simulink model "cla64bit"  (R2020a)
settings: Solver=VariableStepAuto  StartTime=0.0  StopTime=10.0  RelTol=1e-3
(part 1 of 3)
settings Model: Creator=kishan  LastModifiedBy=kishan

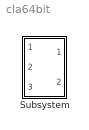
== system cla64bit ==
  Subsystem : Subsystem

== system cla64bit/Subsystem ==
  In1 : Inport
  In3 : Inport  Port=2
  In2 : Inport  Port=3
  Demux : Demux  Outputs=2
  Demux1 : Demux  Outputs=2
  Mux : Mux  Inputs=2
  Subsystem1 : Subsystem
  Subsystem8 : Subsystem
  Out1 : Outport
  Out2 : Outport  Port=2
  wires:
  In1/1 -> Demux/1
  Subsystem8/1(Out1) -> Subsystem1/2(In1)
  Demux1/1 -> Subsystem1/3(In3)
  Mux/1 -> Out2/1
  Subsystem1/1(Out1) -> Out1/1
  Subsystem8/2(Out2) -> Mux/2
  Demux/1 -> Subsystem1/1(In2)
  Demux/2 -> Subsystem8/1(In2)
  Demux1/2 -> Subsystem8/3(In3)
  Subsystem1/2(Out2) -> Mux/1
  In3/1 -> Subsystem8/2(In1)
  In2/1 -> Demux1/1

== system cla64bit/Subsystem/Subsystem1 ==
  In2 : Inport
  In1 : Inport  Port=2
  In3 : Inport  Port=3
  Demux : Demux  Outputs=32
  Demux1 : Demux  Outputs=32
  Mux : Mux  Inputs=32
  Subsystem : Subsystem
  Subsystem1 : Subsystem
  Subsystem2 : Subsystem
  Subsystem3 : Subsystem
  Subsystem4 : Subsystem
  Subsystem5 : Subsystem
  Subsystem6 : Subsystem
  Subsystem7 : Subsystem
  Out1 : Outport
  Out2 : Outport  Port=2
  wires:
  Demux1/30 -> Subsystem/7(In7)
  Demux/11 -> Subsystem5/3(In3)
  Subsystem4/4(Out4) -> Mux/15
  Demux/29 -> Subsystem/1(In1)
  Demux1/4 -> Subsystem7/9(In9)
  Demux/14 -> Subsystem4/2(In2)
  Subsystem/2(Out2) -> Mux/29
  Subsystem7/4(Out4) -> Mux/3
  Subsystem2/3(Out3) -> Mux/22
  Demux/26 -> Subsystem1/2(In2)
  Subsystem7/1(Out1) -> Out1/1
  Subsystem7/3(Out3) -> Mux/2
  Demux/3 -> Subsystem7/3(In3)
  Demux/15 -> Subsystem4/3(In3)
  Subsystem6/1(Out1) -> Subsystem7/5(In5)
  In3/1 -> Demux1/1
  Demux1/31 -> Subsystem/8(In8)
  Demux/20 -> Subsystem3/4(In4)
  Subsystem4/5(Out5) -> Mux/16
  Demux/19 -> Subsystem3/3(In3)
  Subsystem3/5(Out5) -> Mux/20
  Demux1/22 -> Subsystem2/7(In7)
  Subsystem4/3(Out3) -> Mux/14
  Subsystem1/2(Out2) -> Mux/25
  Demux1/15 -> Subsystem4/8(In8)
  Subsystem/4(Out4) -> Mux/31
  Demux/24 -> Subsystem2/4(In4)
  Subsystem5/4(Out4) -> Mux/11
  Subsystem3/3(Out3) -> Mux/18
  Subsystem5/1(Out1) -> Subsystem6/5(In5)
  Subsystem2/2(Out2) -> Mux/21
  Subsystem5/3(Out3) -> Mux/10
  Demux1/16 -> Subsystem4/9(In9)
  Demux/9 -> Subsystem5/1(In1)
  Subsystem7/5(Out5) -> Mux/4
  Demux1/3 -> Subsystem7/8(In8)
  Demux1/29 -> Subsystem/6(In6)
  Demux1/9 -> Subsystem5/6(In6)
  Subsystem2/1(Out1) -> Subsystem3/5(In5)
  Subsystem6/5(Out5) -> Mux/8
  Demux1/25 -> Subsystem1/6(In6)
  Demux/1 -> Subsystem7/1(In1)
  Demux1/13 -> Subsystem4/6(In6)
  Demux/5 -> Subsystem6/1(In1)
  Demux1/7 -> Subsystem6/8(In8)
  Demux1/20 -> Subsystem3/9(In9)
  Subsystem1/4(Out4) -> Mux/27
  In2/1 -> Demux/1
  Demux1/12 -> Subsystem5/9(In9)
  Demux1/18 -> Subsystem3/7(In7)
  Demux/22 -> Subsystem2/2(In2)
  Demux1/32 -> Subsystem/9(In9)
  Subsystem2/4(Out4) -> Mux/23
  Subsystem6/4(Out4) -> Mux/7
  Subsystem5/5(Out5) -> Mux/12
  Demux1/23 -> Subsystem2/8(In8)
  Mux/1 -> Out2/1
  Subsystem6/3(Out3) -> Mux/6
  Demux1/8 -> Subsystem6/9(In9)
  In1/1 -> Subsystem/5(In5)
  Demux/12 -> Subsystem5/4(In4)
  Demux1/17 -> Subsystem3/6(In6)
  Subsystem1/1(Out1) -> Subsystem2/5(In5)
  Subsystem1/5(Out5) -> Mux/28
  Subsystem4/1(Out1) -> Subsystem5/5(In5)
  Demux/6 -> Subsystem6/2(In2)
  Subsystem6/2(Out2) -> Mux/5
  Demux/25 -> Subsystem1/1(In1)
  Subsystem/5(Out5) -> Mux/32
  Subsystem1/3(Out3) -> Mux/26
  Demux1/1 -> Subsystem7/6(In6)
  Demux/31 -> Subsystem/3(In3)
  Demux1/26 -> Subsystem1/7(In7)
  Subsystem/3(Out3) -> Mux/30
  Subsystem3/1(Out1) -> Subsystem4/5(In5)
  Demux/8 -> Subsystem6/4(In4)
  Demux/32 -> Subsystem/4(In4)
  Demux1/19 -> Subsystem3/8(In8)
  Demux1/5 -> Subsystem6/6(In6)
  Subsystem3/4(Out4) -> Mux/19
  Demux/27 -> Subsystem1/3(In3)
  Subsystem/1(Out1) -> Subsystem1/5(In5)
  Demux1/24 -> Subsystem2/9(In9)
  Demux/7 -> Subsystem6/3(In3)
  Demux/30 -> Subsystem/2(In2)
  Demux/4 -> Subsystem7/4(In4)
  Demux/10 -> Subsystem5/2(In2)
  Demux1/28 -> Subsystem1/9(In9)
  Subsystem5/2(Out2) -> Mux/9
  Demux/2 -> Subsystem7/2(In2)
  Demux/17 -> Subsystem3/1(In1)
  Subsystem2/5(Out5) -> Mux/24
  Demux1/6 -> Subsystem6/7(In7)
  Subsystem7/2(Out2) -> Mux/1
  Subsystem4/2(Out2) -> Mux/13
  Demux/13 -> Subsystem4/1(In1)
  Demux/21 -> Subsystem2/1(In1)
  Demux/18 -> Subsystem3/2(In2)
  Subsystem3/2(Out2) -> Mux/17
  Demux1/27 -> Subsystem1/8(In8)
  Demux1/11 -> Subsystem5/8(In8)
  Demux/28 -> Subsystem1/4(In4)
  Demux1/2 -> Subsystem7/7(In7)
  Demux/23 -> Subsystem2/3(In3)
  Demux1/21 -> Subsystem2/6(In6)
  Demux1/14 -> Subsystem4/7(In7)
  Demux/16 -> Subsystem4/4(In4)
  Demux1/10 -> Subsystem5/7(In7)

== system cla64bit/Subsystem/Subsystem8 ==
  In2 : Inport
  In1 : Inport  Port=2
  In3 : Inport  Port=3
  Demux : Demux  Outputs=32
  Demux1 : Demux  Outputs=32
  Mux : Mux  Inputs=32
  Subsystem : Subsystem
  Subsystem1 : Subsystem
  Subsystem2 : Subsystem
  Subsystem3 : Subsystem
  Subsystem4 : Subsystem
  Subsystem5 : Subsystem
  Subsystem6 : Subsystem
  Subsystem7 : Subsystem
  Out1 : Outport
  Out2 : Outport  Port=2
  wires:
  Demux1/30 -> Subsystem/7(In7)
  Demux/11 -> Subsystem5/3(In3)
  Subsystem4/4(Out4) -> Mux/15
  Demux/29 -> Subsystem/1(In1)
  Demux1/4 -> Subsystem7/9(In9)
  Demux/14 -> Subsystem4/2(In2)
  Subsystem/2(Out2) -> Mux/29
  Subsystem7/4(Out4) -> Mux/3
  Subsystem2/3(Out3) -> Mux/22
  Demux/26 -> Subsystem1/2(In2)
  Subsystem7/1(Out1) -> Out1/1
  Subsystem7/3(Out3) -> Mux/2
  Demux/3 -> Subsystem7/3(In3)
  Demux/15 -> Subsystem4/3(In3)
  Subsystem6/1(Out1) -> Subsystem7/5(In5)
  In3/1 -> Demux1/1
  Demux1/31 -> Subsystem/8(In8)
  Demux/20 -> Subsystem3/4(In4)
  Subsystem4/5(Out5) -> Mux/16
  Demux/19 -> Subsystem3/3(In3)
  Subsystem3/5(Out5) -> Mux/20
  Demux1/22 -> Subsystem2/7(In7)
  Subsystem4/3(Out3) -> Mux/14
  Subsystem1/2(Out2) -> Mux/25
  Demux1/15 -> Subsystem4/8(In8)
  Subsystem/4(Out4) -> Mux/31
  Demux/24 -> Subsystem2/4(In4)
  Subsystem5/4(Out4) -> Mux/11
  Subsystem3/3(Out3) -> Mux/18
  Subsystem5/1(Out1) -> Subsystem6/5(In5)
  Subsystem2/2(Out2) -> Mux/21
  Subsystem5/3(Out3) -> Mux/10
  Demux1/16 -> Subsystem4/9(In9)
  Demux/9 -> Subsystem5/1(In1)
  Subsystem7/5(Out5) -> Mux/4
  Demux1/3 -> Subsystem7/8(In8)
  Demux1/29 -> Subsystem/6(In6)
  Demux1/9 -> Subsystem5/6(In6)
  Subsystem2/1(Out1) -> Subsystem3/5(In5)
  Subsystem6/5(Out5) -> Mux/8
  Demux1/25 -> Subsystem1/6(In6)
  Demux/1 -> Subsystem7/1(In1)
  Demux1/13 -> Subsystem4/6(In6)
  Demux/5 -> Subsystem6/1(In1)
  Demux1/7 -> Subsystem6/8(In8)
  Demux1/20 -> Subsystem3/9(In9)
  Subsystem1/4(Out4) -> Mux/27
  In2/1 -> Demux/1
  Demux1/12 -> Subsystem5/9(In9)
  Demux1/18 -> Subsystem3/7(In7)
  Demux/22 -> Subsystem2/2(In2)
  Demux1/32 -> Subsystem/9(In9)
  Subsystem2/4(Out4) -> Mux/23
  Subsystem6/4(Out4) -> Mux/7
  Subsystem5/5(Out5) -> Mux/12
  Demux1/23 -> Subsystem2/8(In8)
  Mux/1 -> Out2/1
  Subsystem6/3(Out3) -> Mux/6
  Demux1/8 -> Subsystem6/9(In9)
  In1/1 -> Subsystem/5(In5)
  Demux/12 -> Subsystem5/4(In4)
  Demux1/17 -> Subsystem3/6(In6)
  Subsystem1/1(Out1) -> Subsystem2/5(In5)
  Subsystem1/5(Out5) -> Mux/28
  Subsystem4/1(Out1) -> Subsystem5/5(In5)
  Demux/6 -> Subsystem6/2(In2)
  Subsystem6/2(Out2) -> Mux/5
  Demux/25 -> Subsystem1/1(In1)
  Subsystem/5(Out5) -> Mux/32
  Subsystem1/3(Out3) -> Mux/26
  Demux1/1 -> Subsystem7/6(In6)
  Demux/31 -> Subsystem/3(In3)
  Demux1/26 -> Subsystem1/7(In7)
  Subsystem/3(Out3) -> Mux/30
  Subsystem3/1(Out1) -> Subsystem4/5(In5)
  Demux/8 -> Subsystem6/4(In4)
  Demux/32 -> Subsystem/4(In4)
  Demux1/19 -> Subsystem3/8(In8)
  Demux1/5 -> Subsystem6/6(In6)
  Subsystem3/4(Out4) -> Mux/19
  Demux/27 -> Subsystem1/3(In3)
  Subsystem/1(Out1) -> Subsystem1/5(In5)
  Demux1/24 -> Subsystem2/9(In9)
  Demux/7 -> Subsystem6/3(In3)
  Demux/30 -> Subsystem/2(In2)
  Demux/4 -> Subsystem7/4(In4)
  Demux/10 -> Subsystem5/2(In2)
  Demux1/28 -> Subsystem1/9(In9)
  Subsystem5/2(Out2) -> Mux/9
  Demux/2 -> Subsystem7/2(In2)
  Demux/17 -> Subsystem3/1(In1)
  Subsystem2/5(Out5) -> Mux/24
  Demux1/6 -> Subsystem6/7(In7)
  Subsystem7/2(Out2) -> Mux/1
  Subsystem4/2(Out2) -> Mux/13
  Demux/13 -> Subsystem4/1(In1)
  Demux/21 -> Subsystem2/1(In1)
  Demux/18 -> Subsystem3/2(In2)
  Subsystem3/2(Out2) -> Mux/17
  Demux1/27 -> Subsystem1/8(In8)
  Demux1/11 -> Subsystem5/8(In8)
  Demux/28 -> Subsystem1/4(In4)
  Demux1/2 -> Subsystem7/7(In7)
  Demux/23 -> Subsystem2/3(In3)
  Demux1/21 -> Subsystem2/6(In6)
  Demux1/14 -> Subsystem4/7(In7)
  Demux/16 -> Subsystem4/4(In4)
  Demux1/10 -> Subsystem5/7(In7)

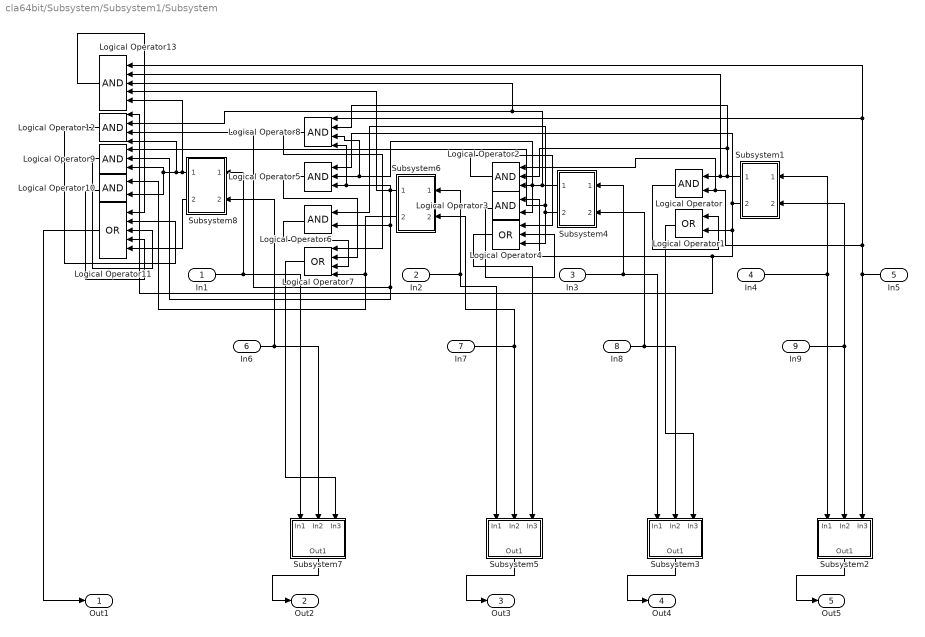
== system cla64bit/Subsystem/Subsystem1/Subsystem ==
  In1 : Inport
  In2 : Inport  Port=2
  In3 : Inport  Port=3
  In4 : Inport  Port=4
  In5 : Inport  Port=5
  In6 : Inport  Port=6
  In7 : Inport  Port=7
  In8 : Inport  Port=8
  In9 : Inport  Port=9
  Logical Operator{,3,6,10} (4 alike) : Logic  AllPortsSameDT=off  OutDataTypeStr=boolean
  Logical Operator1 : Logic  Operator=OR  AllPortsSameDT=off  OutDataTypeStr=boolean
  Logical Operator11 : Logic  Operator=OR  Inputs=5  AllPortsSameDT=off  OutDataTypeStr=boolean
  Logical Operator12 : Logic  Inputs=4  AllPortsSameDT=off  OutDataTypeStr=boolean
  Logical Operator13 : Logic  Inputs=5  AllPortsSameDT=off  OutDataTypeStr=boolean
  Logical Operator2 : Logic  Inputs=3  AllPortsSameDT=off  OutDataTypeStr=boolean
  Logical Operator4 : Logic  Operator=OR  Inputs=3  AllPortsSameDT=off  OutDataTypeStr=boolean
  Logical Operator5 : Logic  Inputs=3  AllPortsSameDT=off  OutDataTypeStr=boolean
  Logical Operator7 : Logic  Operator=OR  Inputs=4  AllPortsSameDT=off  OutDataTypeStr=boolean
  Logical Operator8 : Logic  Inputs=4  AllPortsSameDT=off  OutDataTypeStr=boolean
  Logical Operator9 : Logic  Inputs=3  AllPortsSameDT=off  OutDataTypeStr=boolean
  Subsystem1 : Subsystem
  Subsystem2 : Subsystem
  Subsystem3 : Subsystem
  Subsystem4 : Subsystem
  Subsystem5 : Subsystem
  Subsystem6 : Subsystem
  Subsystem7 : Subsystem
  Subsystem8 : Subsystem
  Out1 : Outport
  Out2 : Outport  Port=2
  Out3 : Outport  Port=3
  Out4 : Outport  Port=4
  Out5 : Outport  Port=5
  wires:
  Subsystem8/2(Out2) -> Logical Operator11/5
  Subsystem5/1(Out1) -> Out3/1
  Logical Operator8/1 -> Logical Operator7/1
  Logical Operator9/1 -> Logical Operator11/3
  Logical Operator5/1 -> Logical Operator7/2
  Logical Operator10/1 -> Logical Operator11/4
  Logical Operator3/1 -> Logical Operator4/2
  Logical Operator/1 -> Logical Operator1/1
  In3/1 -> Subsystem3/1(In1), Subsystem4/1(In1)
  Subsystem6/2(Out2) -> Logical Operator10/1, Logical Operator7/4
  Logical Operator12/1 -> Logical Operator11/2
  In7/1 -> Subsystem5/2(In2), Subsystem6/2(In2)
  Subsystem2/1(Out1) -> Out5/1
  In1/1 -> Subsystem8/1(In1), Subsystem7/1(In1)
  In6/1 -> Subsystem7/2(In2), Subsystem8/2(In2)
  Subsystem1/1(Out1) -> Logical Operator8/2, Logical Operator2/2, Logical Operator13/2, Logical Operator/1
  In9/1 -> Subsystem2/2(In2), Subsystem1/2(In2)
  In8/1 -> Subsystem3/2(In2), Subsystem4/2(In2)
  Logical Operator11/1 -> Out1/1
  Logical Operator2/1 -> Logical Operator4/1
  Subsystem4/1(Out1) -> Logical Operator8/3, Logical Operator5/2, Logical Operator3/2, Logical Operator2/3, Logical Operator13/3, Logical Operator12/2
  Logical Operator13/1 -> Logical Operator11/1
  Subsystem3/1(Out1) -> Out4/1
  In2/1 -> Subsystem6/1(In1), Subsystem5/1(In1)
  Logical Operator6/1 -> Logical Operator7/3
  Subsystem6/1(Out1) -> Logical Operator13/4, Logical Operator12/3, Logical Operator9/2, Logical Operator6/2, Logical Operator8/4, Logical Operator5/3
  Logical Operator7/1 -> Subsystem7/3(In3)
  Subsystem1/2(Out2) -> Logical Operator12/1, Logical Operator3/1, Logical Operator1/2, Logical Operator5/1
  In5/1 -> Subsystem2/3(In3), Logical Operator13/1, Logical Operator8/1, Logical Operator2/1, Logical Operator/2
  In4/1 -> Subsystem2/1(In1), Subsystem1/1(In1)
  Subsystem8/1(Out1) -> Logical Operator13/5, Logical Operator12/4, Logical Operator10/2, Logical Operator9/3
  Subsystem7/1(Out1) -> Out2/1
  Subsystem4/2(Out2) -> Logical Operator9/1, Logical Operator6/1, Logical Operator4/3
  Logical Operator4/1 -> Subsystem5/3(In3)
  Logical Operator1/1 -> Subsystem3/3(In3)

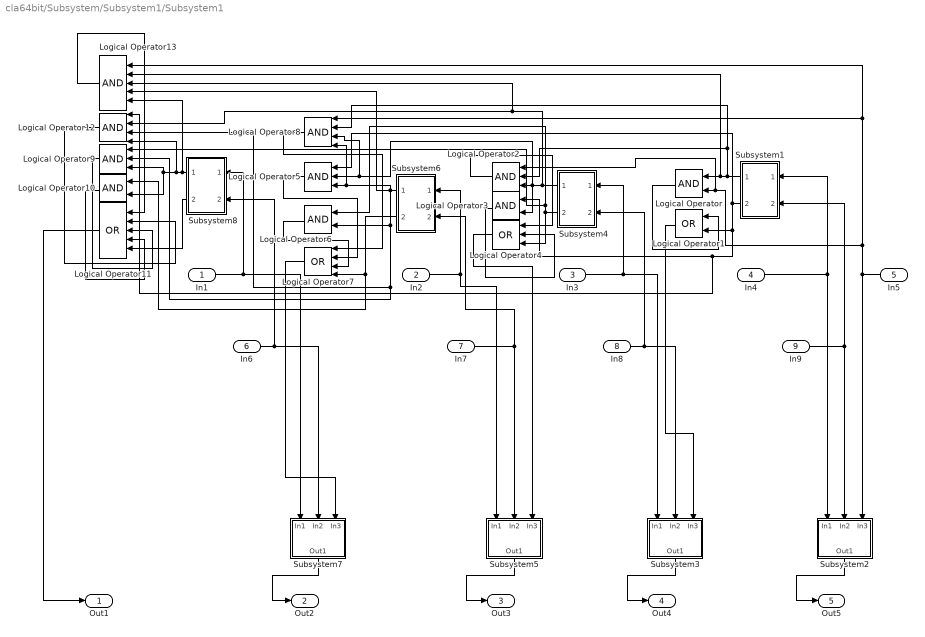
== system cla64bit/Subsystem/Subsystem1/Subsystem1 ==
  In1 : Inport
  In2 : Inport  Port=2
  In3 : Inport  Port=3
  In4 : Inport  Port=4
  In5 : Inport  Port=5
  In6 : Inport  Port=6
  In7 : Inport  Port=7
  In8 : Inport  Port=8
  In9 : Inport  Port=9
  Logical Operator{,3,6,10} (4 alike) : Logic  AllPortsSameDT=off  OutDataTypeStr=boolean
  Logical Operator1 : Logic  Operator=OR  AllPortsSameDT=off  OutDataTypeStr=boolean
  Logical Operator11 : Logic  Operator=OR  Inputs=5  AllPortsSameDT=off  OutDataTypeStr=boolean
  Logical Operator12 : Logic  Inputs=4  AllPortsSameDT=off  OutDataTypeStr=boolean
  Logical Operator13 : Logic  Inputs=5  AllPortsSameDT=off  OutDataTypeStr=boolean
  Logical Operator2 : Logic  Inputs=3  AllPortsSameDT=off  OutDataTypeStr=boolean
  Logical Operator4 : Logic  Operator=OR  Inputs=3  AllPortsSameDT=off  OutDataTypeStr=boolean
  Logical Operator5 : Logic  Inputs=3  AllPortsSameDT=off  OutDataTypeStr=boolean
  Logical Operator7 : Logic  Operator=OR  Inputs=4  AllPortsSameDT=off  OutDataTypeStr=boolean
  Logical Operator8 : Logic  Inputs=4  AllPortsSameDT=off  OutDataTypeStr=boolean
  Logical Operator9 : Logic  Inputs=3  AllPortsSameDT=off  OutDataTypeStr=boolean
  Subsystem1 : Subsystem
  Subsystem2 : Subsystem
  Subsystem3 : Subsystem
  Subsystem4 : Subsystem
  Subsystem5 : Subsystem
  Subsystem6 : Subsystem
  Subsystem7 : Subsystem
  Subsystem8 : Subsystem
  Out1 : Outport
  Out2 : Outport  Port=2
  Out3 : Outport  Port=3
  Out4 : Outport  Port=4
  Out5 : Outport  Port=5
  wires:
  Subsystem8/2(Out2) -> Logical Operator11/5
  Subsystem5/1(Out1) -> Out3/1
  Logical Operator8/1 -> Logical Operator7/1
  Logical Operator9/1 -> Logical Operator11/3
  Logical Operator5/1 -> Logical Operator7/2
  Logical Operator10/1 -> Logical Operator11/4
  Logical Operator3/1 -> Logical Operator4/2
  Logical Operator/1 -> Logical Operator1/1
  In3/1 -> Subsystem3/1(In1), Subsystem4/1(In1)
  Subsystem6/2(Out2) -> Logical Operator10/1, Logical Operator7/4
  Logical Operator12/1 -> Logical Operator11/2
  In7/1 -> Subsystem5/2(In2), Subsystem6/2(In2)
  Subsystem2/1(Out1) -> Out5/1
  In1/1 -> Subsystem8/1(In1), Subsystem7/1(In1)
  In6/1 -> Subsystem7/2(In2), Subsystem8/2(In2)
  Subsystem1/1(Out1) -> Logical Operator8/2, Logical Operator2/2, Logical Operator13/2, Logical Operator/1
  In9/1 -> Subsystem2/2(In2), Subsystem1/2(In2)
  In8/1 -> Subsystem3/2(In2), Subsystem4/2(In2)
  Logical Operator11/1 -> Out1/1
  Logical Operator2/1 -> Logical Operator4/1
  Subsystem4/1(Out1) -> Logical Operator8/3, Logical Operator5/2, Logical Operator3/2, Logical Operator2/3, Logical Operator13/3, Logical Operator12/2
  Logical Operator13/1 -> Logical Operator11/1
  Subsystem3/1(Out1) -> Out4/1
  In2/1 -> Subsystem6/1(In1), Subsystem5/1(In1)
  Logical Operator6/1 -> Logical Operator7/3
  Subsystem6/1(Out1) -> Logical Operator13/4, Logical Operator12/3, Logical Operator9/2, Logical Operator6/2, Logical Operator8/4, Logical Operator5/3
  Logical Operator7/1 -> Subsystem7/3(In3)
  Subsystem1/2(Out2) -> Logical Operator12/1, Logical Operator3/1, Logical Operator1/2, Logical Operator5/1
  In5/1 -> Subsystem2/3(In3), Logical Operator13/1, Logical Operator8/1, Logical Operator2/1, Logical Operator/2
  In4/1 -> Subsystem2/1(In1), Subsystem1/1(In1)
  Subsystem8/1(Out1) -> Logical Operator13/5, Logical Operator12/4, Logical Operator10/2, Logical Operator9/3
  Subsystem7/1(Out1) -> Out2/1
  Subsystem4/2(Out2) -> Logical Operator9/1, Logical Operator6/1, Logical Operator4/3
  Logical Operator4/1 -> Subsystem5/3(In3)
  Logical Operator1/1 -> Subsystem3/3(In3)

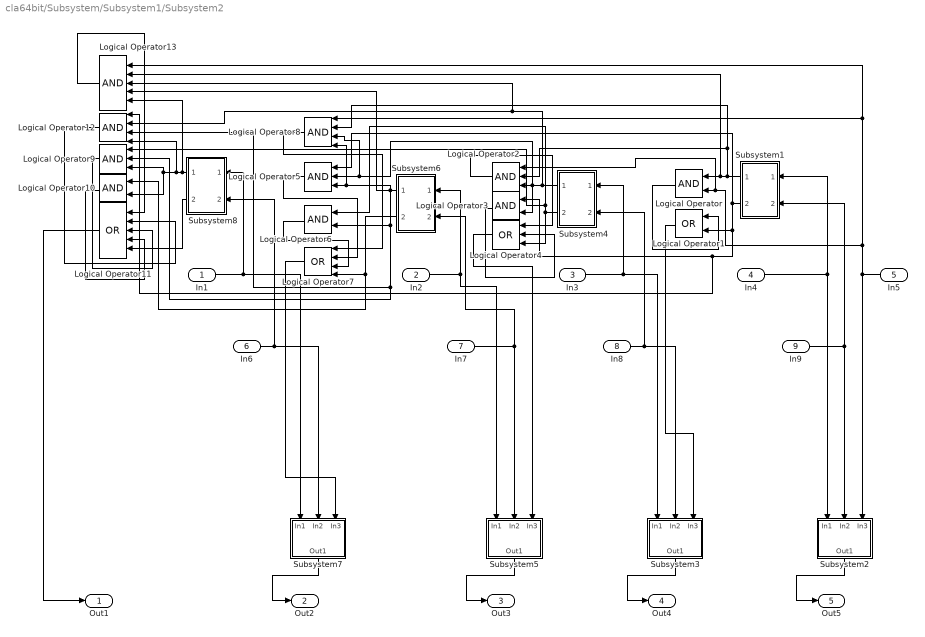
== system cla64bit/Subsystem/Subsystem1/Subsystem2 ==
  In1 : Inport
  In2 : Inport  Port=2
  In3 : Inport  Port=3
  In4 : Inport  Port=4
  In5 : Inport  Port=5
  In6 : Inport  Port=6
  In7 : Inport  Port=7
  In8 : Inport  Port=8
  In9 : Inport  Port=9
  Logical Operator{,3,6,10} (4 alike) : Logic  AllPortsSameDT=off  OutDataTypeStr=boolean
  Logical Operator1 : Logic  Operator=OR  AllPortsSameDT=off  OutDataTypeStr=boolean
  Logical Operator11 : Logic  Operator=OR  Inputs=5  AllPortsSameDT=off  OutDataTypeStr=boolean
  Logical Operator12 : Logic  Inputs=4  AllPortsSameDT=off  OutDataTypeStr=boolean
  Logical Operator13 : Logic  Inputs=5  AllPortsSameDT=off  OutDataTypeStr=boolean
  Logical Operator2 : Logic  Inputs=3  AllPortsSameDT=off  OutDataTypeStr=boolean
  Logical Operator4 : Logic  Operator=OR  Inputs=3  AllPortsSameDT=off  OutDataTypeStr=boolean
  Logical Operator5 : Logic  Inputs=3  AllPortsSameDT=off  OutDataTypeStr=boolean
  Logical Operator7 : Logic  Operator=OR  Inputs=4  AllPortsSameDT=off  OutDataTypeStr=boolean
  Logical Operator8 : Logic  Inputs=4  AllPortsSameDT=off  OutDataTypeStr=boolean
  Logical Operator9 : Logic  Inputs=3  AllPortsSameDT=off  OutDataTypeStr=boolean
  Subsystem1 : Subsystem
  Subsystem2 : Subsystem
  Subsystem3 : Subsystem
  Subsystem4 : Subsystem
  Subsystem5 : Subsystem
  Subsystem6 : Subsystem
  Subsystem7 : Subsystem
  Subsystem8 : Subsystem
  Out1 : Outport
  Out2 : Outport  Port=2
  Out3 : Outport  Port=3
  Out4 : Outport  Port=4
  Out5 : Outport  Port=5
  wires:
  Subsystem8/2(Out2) -> Logical Operator11/5
  Subsystem5/1(Out1) -> Out3/1
  Logical Operator8/1 -> Logical Operator7/1
  Logical Operator9/1 -> Logical Operator11/3
  Logical Operator5/1 -> Logical Operator7/2
  Logical Operator10/1 -> Logical Operator11/4
  Logical Operator3/1 -> Logical Operator4/2
  Logical Operator/1 -> Logical Operator1/1
  In3/1 -> Subsystem3/1(In1), Subsystem4/1(In1)
  Subsystem6/2(Out2) -> Logical Operator10/1, Logical Operator7/4
  Logical Operator12/1 -> Logical Operator11/2
  In7/1 -> Subsystem5/2(In2), Subsystem6/2(In2)
  Subsystem2/1(Out1) -> Out5/1
  In1/1 -> Subsystem8/1(In1), Subsystem7/1(In1)
  In6/1 -> Subsystem7/2(In2), Subsystem8/2(In2)
  Subsystem1/1(Out1) -> Logical Operator8/2, Logical Operator2/2, Logical Operator13/2, Logical Operator/1
  In9/1 -> Subsystem2/2(In2), Subsystem1/2(In2)
  In8/1 -> Subsystem3/2(In2), Subsystem4/2(In2)
  Logical Operator11/1 -> Out1/1
  Logical Operator2/1 -> Logical Operator4/1
  Subsystem4/1(Out1) -> Logical Operator8/3, Logical Operator5/2, Logical Operator3/2, Logical Operator2/3, Logical Operator13/3, Logical Operator12/2
  Logical Operator13/1 -> Logical Operator11/1
  Subsystem3/1(Out1) -> Out4/1
  In2/1 -> Subsystem6/1(In1), Subsystem5/1(In1)
  Logical Operator6/1 -> Logical Operator7/3
  Subsystem6/1(Out1) -> Logical Operator13/4, Logical Operator12/3, Logical Operator9/2, Logical Operator6/2, Logical Operator8/4, Logical Operator5/3
  Logical Operator7/1 -> Subsystem7/3(In3)
  Subsystem1/2(Out2) -> Logical Operator12/1, Logical Operator3/1, Logical Operator1/2, Logical Operator5/1
  In5/1 -> Subsystem2/3(In3), Logical Operator13/1, Logical Operator8/1, Logical Operator2/1, Logical Operator/2
  In4/1 -> Subsystem2/1(In1), Subsystem1/1(In1)
  Subsystem8/1(Out1) -> Logical Operator13/5, Logical Operator12/4, Logical Operator10/2, Logical Operator9/3
  Subsystem7/1(Out1) -> Out2/1
  Subsystem4/2(Out2) -> Logical Operator9/1, Logical Operator6/1, Logical Operator4/3
  Logical Operator4/1 -> Subsystem5/3(In3)
  Logical Operator1/1 -> Subsystem3/3(In3)

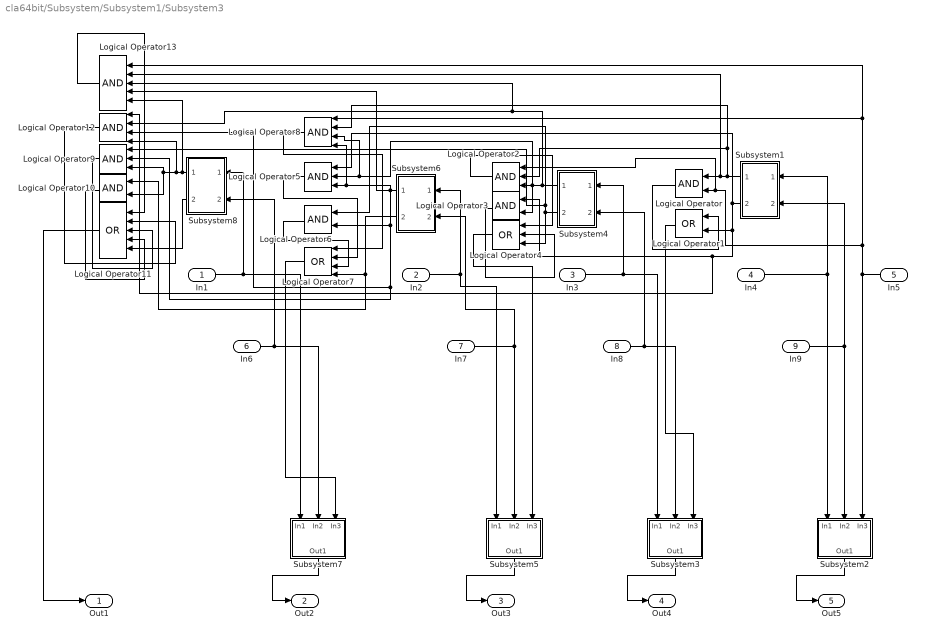
== system cla64bit/Subsystem/Subsystem1/Subsystem3 ==
  In1 : Inport
  In2 : Inport  Port=2
  In3 : Inport  Port=3
  In4 : Inport  Port=4
  In5 : Inport  Port=5
  In6 : Inport  Port=6
  In7 : Inport  Port=7
  In8 : Inport  Port=8
  In9 : Inport  Port=9
  Logical Operator{,3,6,10} (4 alike) : Logic  AllPortsSameDT=off  OutDataTypeStr=boolean
  Logical Operator1 : Logic  Operator=OR  AllPortsSameDT=off  OutDataTypeStr=boolean
  Logical Operator11 : Logic  Operator=OR  Inputs=5  AllPortsSameDT=off  OutDataTypeStr=boolean
  Logical Operator12 : Logic  Inputs=4  AllPortsSameDT=off  OutDataTypeStr=boolean
  Logical Operator13 : Logic  Inputs=5  AllPortsSameDT=off  OutDataTypeStr=boolean
  Logical Operator2 : Logic  Inputs=3  AllPortsSameDT=off  OutDataTypeStr=boolean
  Logical Operator4 : Logic  Operator=OR  Inputs=3  AllPortsSameDT=off  OutDataTypeStr=boolean
  Logical Operator5 : Logic  Inputs=3  AllPortsSameDT=off  OutDataTypeStr=boolean
  Logical Operator7 : Logic  Operator=OR  Inputs=4  AllPortsSameDT=off  OutDataTypeStr=boolean
  Logical Operator8 : Logic  Inputs=4  AllPortsSameDT=off  OutDataTypeStr=boolean
  Logical Operator9 : Logic  Inputs=3  AllPortsSameDT=off  OutDataTypeStr=boolean
  Subsystem1 : Subsystem
  Subsystem2 : Subsystem
  Subsystem3 : Subsystem
  Subsystem4 : Subsystem
  Subsystem5 : Subsystem
  Subsystem6 : Subsystem
  Subsystem7 : Subsystem
  Subsystem8 : Subsystem
  Out1 : Outport
  Out2 : Outport  Port=2
  Out3 : Outport  Port=3
  Out4 : Outport  Port=4
  Out5 : Outport  Port=5
  wires:
  Subsystem8/2(Out2) -> Logical Operator11/5
  Subsystem5/1(Out1) -> Out3/1
  Logical Operator8/1 -> Logical Operator7/1
  Logical Operator9/1 -> Logical Operator11/3
  Logical Operator5/1 -> Logical Operator7/2
  Logical Operator10/1 -> Logical Operator11/4
  Logical Operator3/1 -> Logical Operator4/2
  Logical Operator/1 -> Logical Operator1/1
  In3/1 -> Subsystem3/1(In1), Subsystem4/1(In1)
  Subsystem6/2(Out2) -> Logical Operator10/1, Logical Operator7/4
  Logical Operator12/1 -> Logical Operator11/2
  In7/1 -> Subsystem5/2(In2), Subsystem6/2(In2)
  Subsystem2/1(Out1) -> Out5/1
  In1/1 -> Subsystem8/1(In1), Subsystem7/1(In1)
  In6/1 -> Subsystem7/2(In2), Subsystem8/2(In2)
  Subsystem1/1(Out1) -> Logical Operator8/2, Logical Operator2/2, Logical Operator13/2, Logical Operator/1
  In9/1 -> Subsystem2/2(In2), Subsystem1/2(In2)
  In8/1 -> Subsystem3/2(In2), Subsystem4/2(In2)
  Logical Operator11/1 -> Out1/1
  Logical Operator2/1 -> Logical Operator4/1
  Subsystem4/1(Out1) -> Logical Operator8/3, Logical Operator5/2, Logical Operator3/2, Logical Operator2/3, Logical Operator13/3, Logical Operator12/2
  Logical Operator13/1 -> Logical Operator11/1
  Subsystem3/1(Out1) -> Out4/1
  In2/1 -> Subsystem6/1(In1), Subsystem5/1(In1)
  Logical Operator6/1 -> Logical Operator7/3
  Subsystem6/1(Out1) -> Logical Operator13/4, Logical Operator12/3, Logical Operator9/2, Logical Operator6/2, Logical Operator8/4, Logical Operator5/3
  Logical Operator7/1 -> Subsystem7/3(In3)
  Subsystem1/2(Out2) -> Logical Operator12/1, Logical Operator3/1, Logical Operator1/2, Logical Operator5/1
  In5/1 -> Subsystem2/3(In3), Logical Operator13/1, Logical Operator8/1, Logical Operator2/1, Logical Operator/2
  In4/1 -> Subsystem2/1(In1), Subsystem1/1(In1)
  Subsystem8/1(Out1) -> Logical Operator13/5, Logical Operator12/4, Logical Operator10/2, Logical Operator9/3
  Subsystem7/1(Out1) -> Out2/1
  Subsystem4/2(Out2) -> Logical Operator9/1, Logical Operator6/1, Logical Operator4/3
  Logical Operator4/1 -> Subsystem5/3(In3)
  Logical Operator1/1 -> Subsystem3/3(In3)

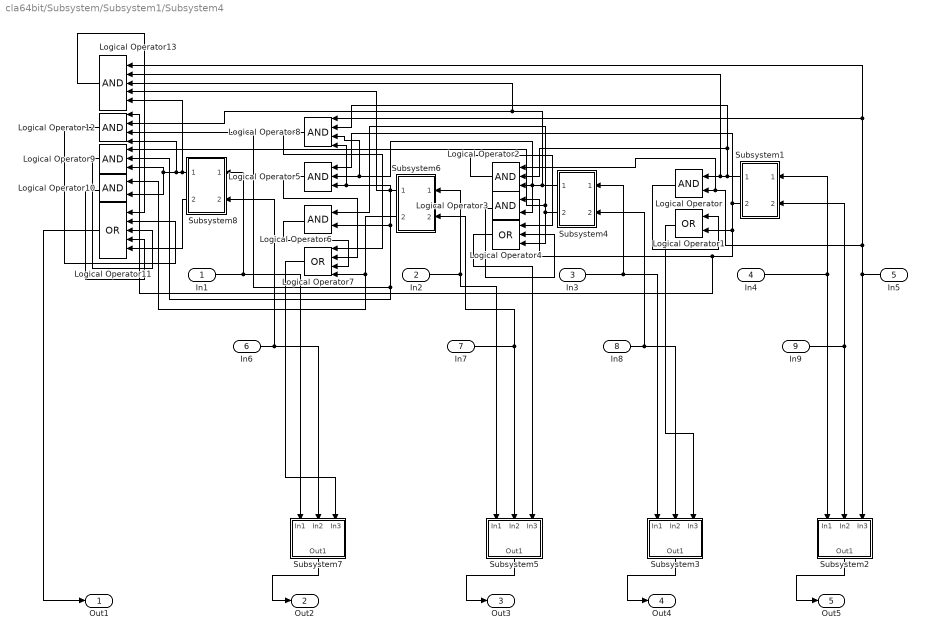
== system cla64bit/Subsystem/Subsystem1/Subsystem4 ==
  In1 : Inport
  In2 : Inport  Port=2
  In3 : Inport  Port=3
  In4 : Inport  Port=4
  In5 : Inport  Port=5
  In6 : Inport  Port=6
  In7 : Inport  Port=7
  In8 : Inport  Port=8
  In9 : Inport  Port=9
  Logical Operator{,3,6,10} (4 alike) : Logic  AllPortsSameDT=off  OutDataTypeStr=boolean
  Logical Operator1 : Logic  Operator=OR  AllPortsSameDT=off  OutDataTypeStr=boolean
  Logical Operator11 : Logic  Operator=OR  Inputs=5  AllPortsSameDT=off  OutDataTypeStr=boolean
  Logical Operator12 : Logic  Inputs=4  AllPortsSameDT=off  OutDataTypeStr=boolean
  Logical Operator13 : Logic  Inputs=5  AllPortsSameDT=off  OutDataTypeStr=boolean
  Logical Operator2 : Logic  Inputs=3  AllPortsSameDT=off  OutDataTypeStr=boolean
  Logical Operator4 : Logic  Operator=OR  Inputs=3  AllPortsSameDT=off  OutDataTypeStr=boolean
  Logical Operator5 : Logic  Inputs=3  AllPortsSameDT=off  OutDataTypeStr=boolean
  Logical Operator7 : Logic  Operator=OR  Inputs=4  AllPortsSameDT=off  OutDataTypeStr=boolean
  Logical Operator8 : Logic  Inputs=4  AllPortsSameDT=off  OutDataTypeStr=boolean
  Logical Operator9 : Logic  Inputs=3  AllPortsSameDT=off  OutDataTypeStr=boolean
  Subsystem1 : Subsystem
  Subsystem2 : Subsystem
  Subsystem3 : Subsystem
  Subsystem4 : Subsystem
  Subsystem5 : Subsystem
  Subsystem6 : Subsystem
  Subsystem7 : Subsystem
  Subsystem8 : Subsystem
  Out1 : Outport
  Out2 : Outport  Port=2
  Out3 : Outport  Port=3
  Out4 : Outport  Port=4
  Out5 : Outport  Port=5
  wires:
  Subsystem8/2(Out2) -> Logical Operator11/5
  Subsystem5/1(Out1) -> Out3/1
  Logical Operator8/1 -> Logical Operator7/1
  Logical Operator9/1 -> Logical Operator11/3
  Logical Operator5/1 -> Logical Operator7/2
  Logical Operator10/1 -> Logical Operator11/4
  Logical Operator3/1 -> Logical Operator4/2
  Logical Operator/1 -> Logical Operator1/1
  In3/1 -> Subsystem3/1(In1), Subsystem4/1(In1)
  Subsystem6/2(Out2) -> Logical Operator10/1, Logical Operator7/4
  Logical Operator12/1 -> Logical Operator11/2
  In7/1 -> Subsystem5/2(In2), Subsystem6/2(In2)
  Subsystem2/1(Out1) -> Out5/1
  In1/1 -> Subsystem8/1(In1), Subsystem7/1(In1)
  In6/1 -> Subsystem7/2(In2), Subsystem8/2(In2)
  Subsystem1/1(Out1) -> Logical Operator8/2, Logical Operator2/2, Logical Operator13/2, Logical Operator/1
  In9/1 -> Subsystem2/2(In2), Subsystem1/2(In2)
  In8/1 -> Subsystem3/2(In2), Subsystem4/2(In2)
  Logical Operator11/1 -> Out1/1
  Logical Operator2/1 -> Logical Operator4/1
  Subsystem4/1(Out1) -> Logical Operator8/3, Logical Operator5/2, Logical Operator3/2, Logical Operator2/3, Logical Operator13/3, Logical Operator12/2
  Logical Operator13/1 -> Logical Operator11/1
  Subsystem3/1(Out1) -> Out4/1
  In2/1 -> Subsystem6/1(In1), Subsystem5/1(In1)
  Logical Operator6/1 -> Logical Operator7/3
  Subsystem6/1(Out1) -> Logical Operator13/4, Logical Operator12/3, Logical Operator9/2, Logical Operator6/2, Logical Operator8/4, Logical Operator5/3
  Logical Operator7/1 -> Subsystem7/3(In3)
  Subsystem1/2(Out2) -> Logical Operator12/1, Logical Operator3/1, Logical Operator1/2, Logical Operator5/1
  In5/1 -> Subsystem2/3(In3), Logical Operator13/1, Logical Operator8/1, Logical Operator2/1, Logical Operator/2
  In4/1 -> Subsystem2/1(In1), Subsystem1/1(In1)
  Subsystem8/1(Out1) -> Logical Operator13/5, Logical Operator12/4, Logical Operator10/2, Logical Operator9/3
  Subsystem7/1(Out1) -> Out2/1
  Subsystem4/2(Out2) -> Logical Operator9/1, Logical Operator6/1, Logical Operator4/3
  Logical Operator4/1 -> Subsystem5/3(In3)
  Logical Operator1/1 -> Subsystem3/3(In3)

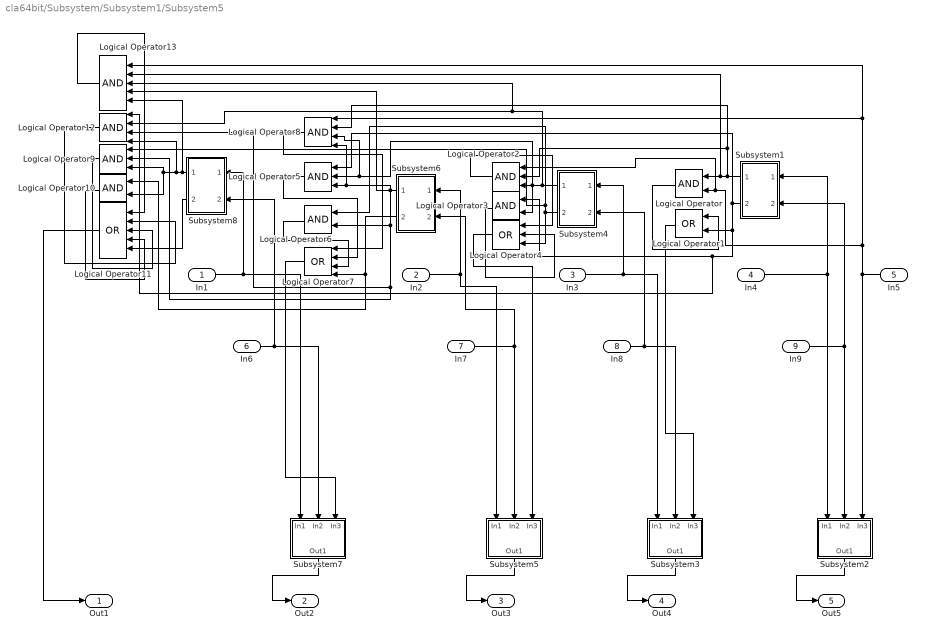
== system cla64bit/Subsystem/Subsystem1/Subsystem5 ==
  In1 : Inport
  In2 : Inport  Port=2
  In3 : Inport  Port=3
  In4 : Inport  Port=4
  In5 : Inport  Port=5
  In6 : Inport  Port=6
  In7 : Inport  Port=7
  In8 : Inport  Port=8
  In9 : Inport  Port=9
  Logical Operator{,3,6,10} (4 alike) : Logic  AllPortsSameDT=off  OutDataTypeStr=boolean
  Logical Operator1 : Logic  Operator=OR  AllPortsSameDT=off  OutDataTypeStr=boolean
  Logical Operator11 : Logic  Operator=OR  Inputs=5  AllPortsSameDT=off  OutDataTypeStr=boolean
  Logical Operator12 : Logic  Inputs=4  AllPortsSameDT=off  OutDataTypeStr=boolean
  Logical Operator13 : Logic  Inputs=5  AllPortsSameDT=off  OutDataTypeStr=boolean
  Logical Operator2 : Logic  Inputs=3  AllPortsSameDT=off  OutDataTypeStr=boolean
  Logical Operator4 : Logic  Operator=OR  Inputs=3  AllPortsSameDT=off  OutDataTypeStr=boolean
  Logical Operator5 : Logic  Inputs=3  AllPortsSameDT=off  OutDataTypeStr=boolean
  Logical Operator7 : Logic  Operator=OR  Inputs=4  AllPortsSameDT=off  OutDataTypeStr=boolean
  Logical Operator8 : Logic  Inputs=4  AllPortsSameDT=off  OutDataTypeStr=boolean
  Logical Operator9 : Logic  Inputs=3  AllPortsSameDT=off  OutDataTypeStr=boolean
  Subsystem1 : Subsystem
  Subsystem2 : Subsystem
  Subsystem3 : Subsystem
  Subsystem4 : Subsystem
  Subsystem5 : Subsystem
  Subsystem6 : Subsystem
  Subsystem7 : Subsystem
  Subsystem8 : Subsystem
  Out1 : Outport
  Out2 : Outport  Port=2
  Out3 : Outport  Port=3
  Out4 : Outport  Port=4
  Out5 : Outport  Port=5
  wires:
  Subsystem8/2(Out2) -> Logical Operator11/5
  Subsystem5/1(Out1) -> Out3/1
  Logical Operator8/1 -> Logical Operator7/1
  Logical Operator9/1 -> Logical Operator11/3
  Logical Operator5/1 -> Logical Operator7/2
  Logical Operator10/1 -> Logical Operator11/4
  Logical Operator3/1 -> Logical Operator4/2
  Logical Operator/1 -> Logical Operator1/1
  In3/1 -> Subsystem3/1(In1), Subsystem4/1(In1)
  Subsystem6/2(Out2) -> Logical Operator10/1, Logical Operator7/4
  Logical Operator12/1 -> Logical Operator11/2
  In7/1 -> Subsystem5/2(In2), Subsystem6/2(In2)
  Subsystem2/1(Out1) -> Out5/1
  In1/1 -> Subsystem8/1(In1), Subsystem7/1(In1)
  In6/1 -> Subsystem7/2(In2), Subsystem8/2(In2)
  Subsystem1/1(Out1) -> Logical Operator8/2, Logical Operator2/2, Logical Operator13/2, Logical Operator/1
  In9/1 -> Subsystem2/2(In2), Subsystem1/2(In2)
  In8/1 -> Subsystem3/2(In2), Subsystem4/2(In2)
  Logical Operator11/1 -> Out1/1
  Logical Operator2/1 -> Logical Operator4/1
  Subsystem4/1(Out1) -> Logical Operator8/3, Logical Operator5/2, Logical Operator3/2, Logical Operator2/3, Logical Operator13/3, Logical Operator12/2
  Logical Operator13/1 -> Logical Operator11/1
  Subsystem3/1(Out1) -> Out4/1
  In2/1 -> Subsystem6/1(In1), Subsystem5/1(In1)
  Logical Operator6/1 -> Logical Operator7/3
  Subsystem6/1(Out1) -> Logical Operator13/4, Logical Operator12/3, Logical Operator9/2, Logical Operator6/2, Logical Operator8/4, Logical Operator5/3
  Logical Operator7/1 -> Subsystem7/3(In3)
  Subsystem1/2(Out2) -> Logical Operator12/1, Logical Operator3/1, Logical Operator1/2, Logical Operator5/1
  In5/1 -> Subsystem2/3(In3), Logical Operator13/1, Logical Operator8/1, Logical Operator2/1, Logical Operator/2
  In4/1 -> Subsystem2/1(In1), Subsystem1/1(In1)
  Subsystem8/1(Out1) -> Logical Operator13/5, Logical Operator12/4, Logical Operator10/2, Logical Operator9/3
  Subsystem7/1(Out1) -> Out2/1
  Subsystem4/2(Out2) -> Logical Operator9/1, Logical Operator6/1, Logical Operator4/3
  Logical Operator4/1 -> Subsystem5/3(In3)
  Logical Operator1/1 -> Subsystem3/3(In3)

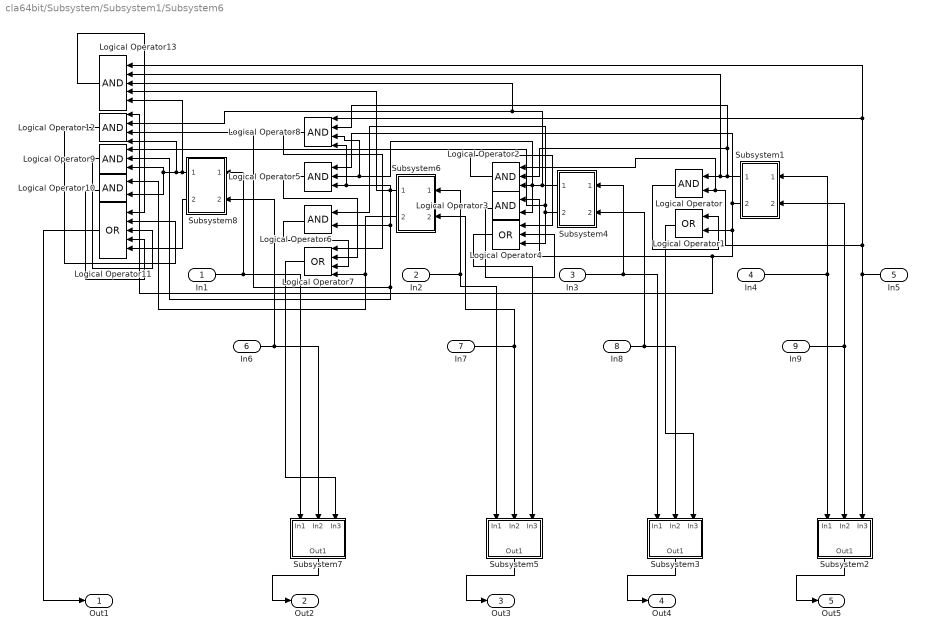
== system cla64bit/Subsystem/Subsystem1/Subsystem6 ==
  In1 : Inport
  In2 : Inport  Port=2
  In3 : Inport  Port=3
  In4 : Inport  Port=4
  In5 : Inport  Port=5
  In6 : Inport  Port=6
  In7 : Inport  Port=7
  In8 : Inport  Port=8
  In9 : Inport  Port=9
  Logical Operator{,3,6,10} (4 alike) : Logic  AllPortsSameDT=off  OutDataTypeStr=boolean
  Logical Operator1 : Logic  Operator=OR  AllPortsSameDT=off  OutDataTypeStr=boolean
  Logical Operator11 : Logic  Operator=OR  Inputs=5  AllPortsSameDT=off  OutDataTypeStr=boolean
  Logical Operator12 : Logic  Inputs=4  AllPortsSameDT=off  OutDataTypeStr=boolean
  Logical Operator13 : Logic  Inputs=5  AllPortsSameDT=off  OutDataTypeStr=boolean
  Logical Operator2 : Logic  Inputs=3  AllPortsSameDT=off  OutDataTypeStr=boolean
  Logical Operator4 : Logic  Operator=OR  Inputs=3  AllPortsSameDT=off  OutDataTypeStr=boolean
  Logical Operator5 : Logic  Inputs=3  AllPortsSameDT=off  OutDataTypeStr=boolean
  Logical Operator7 : Logic  Operator=OR  Inputs=4  AllPortsSameDT=off  OutDataTypeStr=boolean
  Logical Operator8 : Logic  Inputs=4  AllPortsSameDT=off  OutDataTypeStr=boolean
  Logical Operator9 : Logic  Inputs=3  AllPortsSameDT=off  OutDataTypeStr=boolean
  Subsystem1 : Subsystem
  Subsystem2 : Subsystem
  Subsystem3 : Subsystem
  Subsystem4 : Subsystem
  Subsystem5 : Subsystem
  Subsystem6 : Subsystem
  Subsystem7 : Subsystem
  Subsystem8 : Subsystem
  Out1 : Outport
  Out2 : Outport  Port=2
  Out3 : Outport  Port=3
  Out4 : Outport  Port=4
  Out5 : Outport  Port=5
  wires:
  Subsystem8/2(Out2) -> Logical Operator11/5
  Subsystem5/1(Out1) -> Out3/1
  Logical Operator8/1 -> Logical Operator7/1
  Logical Operator9/1 -> Logical Operator11/3
  Logical Operator5/1 -> Logical Operator7/2
  Logical Operator10/1 -> Logical Operator11/4
  Logical Operator3/1 -> Logical Operator4/2
  Logical Operator/1 -> Logical Operator1/1
  In3/1 -> Subsystem3/1(In1), Subsystem4/1(In1)
  Subsystem6/2(Out2) -> Logical Operator10/1, Logical Operator7/4
  Logical Operator12/1 -> Logical Operator11/2
  In7/1 -> Subsystem5/2(In2), Subsystem6/2(In2)
  Subsystem2/1(Out1) -> Out5/1
  In1/1 -> Subsystem8/1(In1), Subsystem7/1(In1)
  In6/1 -> Subsystem7/2(In2), Subsystem8/2(In2)
  Subsystem1/1(Out1) -> Logical Operator8/2, Logical Operator2/2, Logical Operator13/2, Logical Operator/1
  In9/1 -> Subsystem2/2(In2), Subsystem1/2(In2)
  In8/1 -> Subsystem3/2(In2), Subsystem4/2(In2)
  Logical Operator11/1 -> Out1/1
  Logical Operator2/1 -> Logical Operator4/1
  Subsystem4/1(Out1) -> Logical Operator8/3, Logical Operator5/2, Logical Operator3/2, Logical Operator2/3, Logical Operator13/3, Logical Operator12/2
  Logical Operator13/1 -> Logical Operator11/1
  Subsystem3/1(Out1) -> Out4/1
  In2/1 -> Subsystem6/1(In1), Subsystem5/1(In1)
  Logical Operator6/1 -> Logical Operator7/3
  Subsystem6/1(Out1) -> Logical Operator13/4, Logical Operator12/3, Logical Operator9/2, Logical Operator6/2, Logical Operator8/4, Logical Operator5/3
  Logical Operator7/1 -> Subsystem7/3(In3)
  Subsystem1/2(Out2) -> Logical Operator12/1, Logical Operator3/1, Logical Operator1/2, Logical Operator5/1
  In5/1 -> Subsystem2/3(In3), Logical Operator13/1, Logical Operator8/1, Logical Operator2/1, Logical Operator/2
  In4/1 -> Subsystem2/1(In1), Subsystem1/1(In1)
  Subsystem8/1(Out1) -> Logical Operator13/5, Logical Operator12/4, Logical Operator10/2, Logical Operator9/3
  Subsystem7/1(Out1) -> Out2/1
  Subsystem4/2(Out2) -> Logical Operator9/1, Logical Operator6/1, Logical Operator4/3
  Logical Operator4/1 -> Subsystem5/3(In3)
  Logical Operator1/1 -> Subsystem3/3(In3)

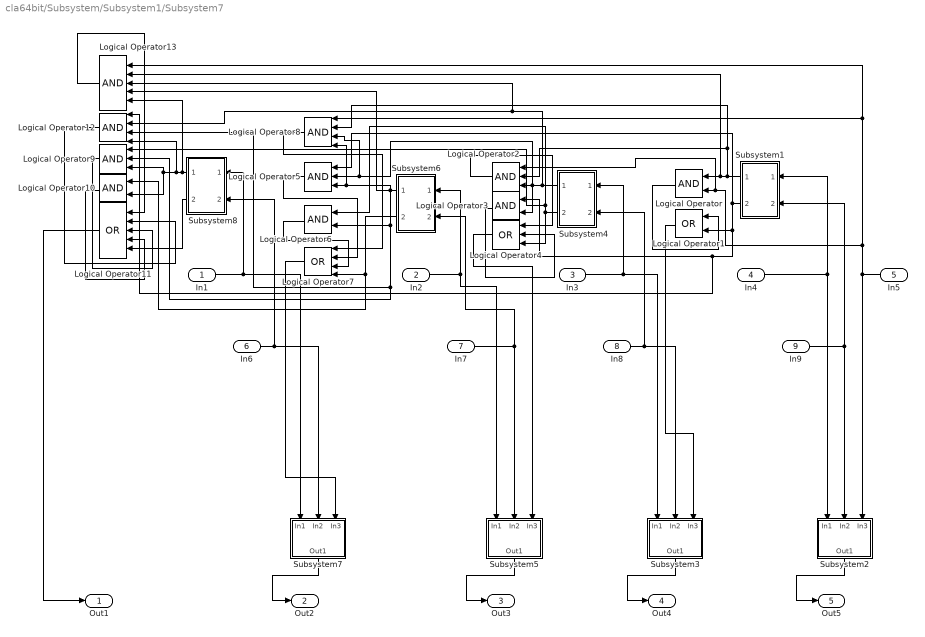
== system cla64bit/Subsystem/Subsystem1/Subsystem7 ==
  In1 : Inport
  In2 : Inport  Port=2
  In3 : Inport  Port=3
  In4 : Inport  Port=4
  In5 : Inport  Port=5
  In6 : Inport  Port=6
  In7 : Inport  Port=7
  In8 : Inport  Port=8
  In9 : Inport  Port=9
  Logical Operator{,3,6,10} (4 alike) : Logic  AllPortsSameDT=off  OutDataTypeStr=boolean
  Logical Operator1 : Logic  Operator=OR  AllPortsSameDT=off  OutDataTypeStr=boolean
  Logical Operator11 : Logic  Operator=OR  Inputs=5  AllPortsSameDT=off  OutDataTypeStr=boolean
  Logical Operator12 : Logic  Inputs=4  AllPortsSameDT=off  OutDataTypeStr=boolean
  Logical Operator13 : Logic  Inputs=5  AllPortsSameDT=off  OutDataTypeStr=boolean
  Logical Operator2 : Logic  Inputs=3  AllPortsSameDT=off  OutDataTypeStr=boolean
  Logical Operator4 : Logic  Operator=OR  Inputs=3  AllPortsSameDT=off  OutDataTypeStr=boolean
  Logical Operator5 : Logic  Inputs=3  AllPortsSameDT=off  OutDataTypeStr=boolean
  Logical Operator7 : Logic  Operator=OR  Inputs=4  AllPortsSameDT=off  OutDataTypeStr=boolean
  Logical Operator8 : Logic  Inputs=4  AllPortsSameDT=off  OutDataTypeStr=boolean
  Logical Operator9 : Logic  Inputs=3  AllPortsSameDT=off  OutDataTypeStr=boolean
  Subsystem1 : Subsystem
  Subsystem2 : Subsystem
  Subsystem3 : Subsystem
  Subsystem4 : Subsystem
  Subsystem5 : Subsystem
  Subsystem6 : Subsystem
  Subsystem7 : Subsystem
  Subsystem8 : Subsystem
  Out1 : Outport
  Out2 : Outport  Port=2
  Out3 : Outport  Port=3
  Out4 : Outport  Port=4
  Out5 : Outport  Port=5
  wires:
  Subsystem8/2(Out2) -> Logical Operator11/5
  Subsystem5/1(Out1) -> Out3/1
  Logical Operator8/1 -> Logical Operator7/1
  Logical Operator9/1 -> Logical Operator11/3
  Logical Operator5/1 -> Logical Operator7/2
  Logical Operator10/1 -> Logical Operator11/4
  Logical Operator3/1 -> Logical Operator4/2
  Logical Operator/1 -> Logical Operator1/1
  In3/1 -> Subsystem3/1(In1), Subsystem4/1(In1)
  Subsystem6/2(Out2) -> Logical Operator10/1, Logical Operator7/4
  Logical Operator12/1 -> Logical Operator11/2
  In7/1 -> Subsystem5/2(In2), Subsystem6/2(In2)
  Subsystem2/1(Out1) -> Out5/1
  In1/1 -> Subsystem8/1(In1), Subsystem7/1(In1)
  In6/1 -> Subsystem7/2(In2), Subsystem8/2(In2)
  Subsystem1/1(Out1) -> Logical Operator8/2, Logical Operator2/2, Logical Operator13/2, Logical Operator/1
  In9/1 -> Subsystem2/2(In2), Subsystem1/2(In2)
  In8/1 -> Subsystem3/2(In2), Subsystem4/2(In2)
  Logical Operator11/1 -> Out1/1
  Logical Operator2/1 -> Logical Operator4/1
  Subsystem4/1(Out1) -> Logical Operator8/3, Logical Operator5/2, Logical Operator3/2, Logical Operator2/3, Logical Operator13/3, Logical Operator12/2
  Logical Operator13/1 -> Logical Operator11/1
  Subsystem3/1(Out1) -> Out4/1
  In2/1 -> Subsystem6/1(In1), Subsystem5/1(In1)
  Logical Operator6/1 -> Logical Operator7/3
  Subsystem6/1(Out1) -> Logical Operator13/4, Logical Operator12/3, Logical Operator9/2, Logical Operator6/2, Logical Operator8/4, Logical Operator5/3
  Logical Operator7/1 -> Subsystem7/3(In3)
  Subsystem1/2(Out2) -> Logical Operator12/1, Logical Operator3/1, Logical Operator1/2, Logical Operator5/1
  In5/1 -> Subsystem2/3(In3), Logical Operator13/1, Logical Operator8/1, Logical Operator2/1, Logical Operator/2
  In4/1 -> Subsystem2/1(In1), Subsystem1/1(In1)
  Subsystem8/1(Out1) -> Logical Operator13/5, Logical Operator12/4, Logical Operator10/2, Logical Operator9/3
  Subsystem7/1(Out1) -> Out2/1
  Subsystem4/2(Out2) -> Logical Operator9/1, Logical Operator6/1, Logical Operator4/3
  Logical Operator4/1 -> Subsystem5/3(In3)
  Logical Operator1/1 -> Subsystem3/3(In3)

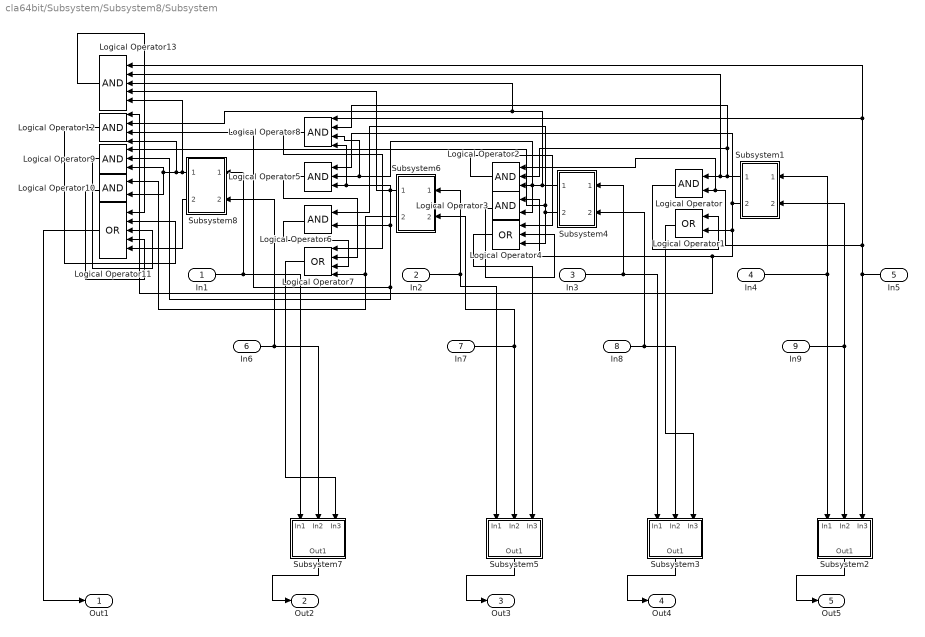
== system cla64bit/Subsystem/Subsystem8/Subsystem ==
  In1 : Inport
  In2 : Inport  Port=2
  In3 : Inport  Port=3
  In4 : Inport  Port=4
  In5 : Inport  Port=5
  In6 : Inport  Port=6
  In7 : Inport  Port=7
  In8 : Inport  Port=8
  In9 : Inport  Port=9
  Logical Operator{,3,6,10} (4 alike) : Logic  AllPortsSameDT=off  OutDataTypeStr=boolean
  Logical Operator1 : Logic  Operator=OR  AllPortsSameDT=off  OutDataTypeStr=boolean
  Logical Operator11 : Logic  Operator=OR  Inputs=5  AllPortsSameDT=off  OutDataTypeStr=boolean
  Logical Operator12 : Logic  Inputs=4  AllPortsSameDT=off  OutDataTypeStr=boolean
  Logical Operator13 : Logic  Inputs=5  AllPortsSameDT=off  OutDataTypeStr=boolean
  Logical Operator2 : Logic  Inputs=3  AllPortsSameDT=off  OutDataTypeStr=boolean
  Logical Operator4 : Logic  Operator=OR  Inputs=3  AllPortsSameDT=off  OutDataTypeStr=boolean
  Logical Operator5 : Logic  Inputs=3  AllPortsSameDT=off  OutDataTypeStr=boolean
  Logical Operator7 : Logic  Operator=OR  Inputs=4  AllPortsSameDT=off  OutDataTypeStr=boolean
  Logical Operator8 : Logic  Inputs=4  AllPortsSameDT=off  OutDataTypeStr=boolean
  Logical Operator9 : Logic  Inputs=3  AllPortsSameDT=off  OutDataTypeStr=boolean
  Subsystem1 : Subsystem
  Subsystem2 : Subsystem
  Subsystem3 : Subsystem
  Subsystem4 : Subsystem
  Subsystem5 : Subsystem
  Subsystem6 : Subsystem
  Subsystem7 : Subsystem
  Subsystem8 : Subsystem
  Out1 : Outport
  Out2 : Outport  Port=2
  Out3 : Outport  Port=3
  Out4 : Outport  Port=4
  Out5 : Outport  Port=5
  wires:
  Subsystem8/2(Out2) -> Logical Operator11/5
  Subsystem5/1(Out1) -> Out3/1
  Logical Operator8/1 -> Logical Operator7/1
  Logical Operator9/1 -> Logical Operator11/3
  Logical Operator5/1 -> Logical Operator7/2
  Logical Operator10/1 -> Logical Operator11/4
  Logical Operator3/1 -> Logical Operator4/2
  Logical Operator/1 -> Logical Operator1/1
  In3/1 -> Subsystem3/1(In1), Subsystem4/1(In1)
  Subsystem6/2(Out2) -> Logical Operator10/1, Logical Operator7/4
  Logical Operator12/1 -> Logical Operator11/2
  In7/1 -> Subsystem5/2(In2), Subsystem6/2(In2)
  Subsystem2/1(Out1) -> Out5/1
  In1/1 -> Subsystem8/1(In1), Subsystem7/1(In1)
  In6/1 -> Subsystem7/2(In2), Subsystem8/2(In2)
  Subsystem1/1(Out1) -> Logical Operator8/2, Logical Operator2/2, Logical Operator13/2, Logical Operator/1
  In9/1 -> Subsystem2/2(In2), Subsystem1/2(In2)
  In8/1 -> Subsystem3/2(In2), Subsystem4/2(In2)
  Logical Operator11/1 -> Out1/1
  Logical Operator2/1 -> Logical Operator4/1
  Subsystem4/1(Out1) -> Logical Operator8/3, Logical Operator5/2, Logical Operator3/2, Logical Operator2/3, Logical Operator13/3, Logical Operator12/2
  Logical Operator13/1 -> Logical Operator11/1
  Subsystem3/1(Out1) -> Out4/1
  In2/1 -> Subsystem6/1(In1), Subsystem5/1(In1)
  Logical Operator6/1 -> Logical Operator7/3
  Subsystem6/1(Out1) -> Logical Operator13/4, Logical Operator12/3, Logical Operator9/2, Logical Operator6/2, Logical Operator8/4, Logical Operator5/3
  Logical Operator7/1 -> Subsystem7/3(In3)
  Subsystem1/2(Out2) -> Logical Operator12/1, Logical Operator3/1, Logical Operator1/2, Logical Operator5/1
  In5/1 -> Subsystem2/3(In3), Logical Operator13/1, Logical Operator8/1, Logical Operator2/1, Logical Operator/2
  In4/1 -> Subsystem2/1(In1), Subsystem1/1(In1)
  Subsystem8/1(Out1) -> Logical Operator13/5, Logical Operator12/4, Logical Operator10/2, Logical Operator9/3
  Subsystem7/1(Out1) -> Out2/1
  Subsystem4/2(Out2) -> Logical Operator9/1, Logical Operator6/1, Logical Operator4/3
  Logical Operator4/1 -> Subsystem5/3(In3)
  Logical Operator1/1 -> Subsystem3/3(In3)

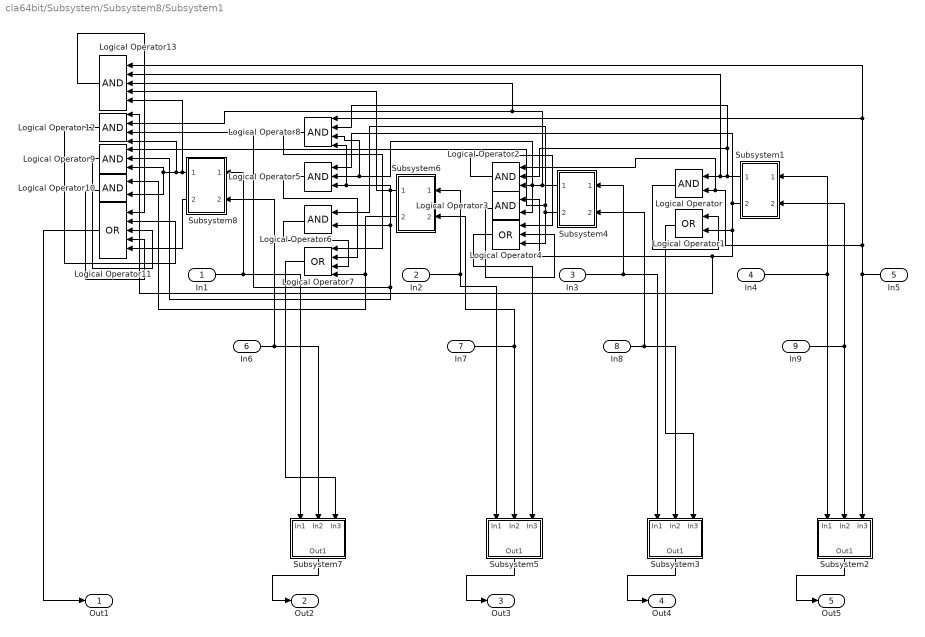
== system cla64bit/Subsystem/Subsystem8/Subsystem1 ==
  In1 : Inport
  In2 : Inport  Port=2
  In3 : Inport  Port=3
  In4 : Inport  Port=4
  In5 : Inport  Port=5
  In6 : Inport  Port=6
  In7 : Inport  Port=7
  In8 : Inport  Port=8
  In9 : Inport  Port=9
  Logical Operator{,3,6,10} (4 alike) : Logic  AllPortsSameDT=off  OutDataTypeStr=boolean
  Logical Operator1 : Logic  Operator=OR  AllPortsSameDT=off  OutDataTypeStr=boolean
  Logical Operator11 : Logic  Operator=OR  Inputs=5  AllPortsSameDT=off  OutDataTypeStr=boolean
  Logical Operator12 : Logic  Inputs=4  AllPortsSameDT=off  OutDataTypeStr=boolean
  Logical Operator13 : Logic  Inputs=5  AllPortsSameDT=off  OutDataTypeStr=boolean
  Logical Operator2 : Logic  Inputs=3  AllPortsSameDT=off  OutDataTypeStr=boolean
  Logical Operator4 : Logic  Operator=OR  Inputs=3  AllPortsSameDT=off  OutDataTypeStr=boolean
  Logical Operator5 : Logic  Inputs=3  AllPortsSameDT=off  OutDataTypeStr=boolean
  Logical Operator7 : Logic  Operator=OR  Inputs=4  AllPortsSameDT=off  OutDataTypeStr=boolean
  Logical Operator8 : Logic  Inputs=4  AllPortsSameDT=off  OutDataTypeStr=boolean
  Logical Operator9 : Logic  Inputs=3  AllPortsSameDT=off  OutDataTypeStr=boolean
  Subsystem1 : Subsystem
  Subsystem2 : Subsystem
  Subsystem3 : Subsystem
  Subsystem4 : Subsystem
  Subsystem5 : Subsystem
  Subsystem6 : Subsystem
  Subsystem7 : Subsystem
  Subsystem8 : Subsystem
  Out1 : Outport
  Out2 : Outport  Port=2
  Out3 : Outport  Port=3
  Out4 : Outport  Port=4
  Out5 : Outport  Port=5
  wires:
  Subsystem8/2(Out2) -> Logical Operator11/5
  Subsystem5/1(Out1) -> Out3/1
  Logical Operator8/1 -> Logical Operator7/1
  Logical Operator9/1 -> Logical Operator11/3
  Logical Operator5/1 -> Logical Operator7/2
  Logical Operator10/1 -> Logical Operator11/4
  Logical Operator3/1 -> Logical Operator4/2
  Logical Operator/1 -> Logical Operator1/1
  In3/1 -> Subsystem3/1(In1), Subsystem4/1(In1)
  Subsystem6/2(Out2) -> Logical Operator10/1, Logical Operator7/4
  Logical Operator12/1 -> Logical Operator11/2
  In7/1 -> Subsystem5/2(In2), Subsystem6/2(In2)
  Subsystem2/1(Out1) -> Out5/1
  In1/1 -> Subsystem8/1(In1), Subsystem7/1(In1)
  In6/1 -> Subsystem7/2(In2), Subsystem8/2(In2)
  Subsystem1/1(Out1) -> Logical Operator8/2, Logical Operator2/2, Logical Operator13/2, Logical Operator/1
  In9/1 -> Subsystem2/2(In2), Subsystem1/2(In2)
  In8/1 -> Subsystem3/2(In2), Subsystem4/2(In2)
  Logical Operator11/1 -> Out1/1
  Logical Operator2/1 -> Logical Operator4/1
  Subsystem4/1(Out1) -> Logical Operator8/3, Logical Operator5/2, Logical Operator3/2, Logical Operator2/3, Logical Operator13/3, Logical Operator12/2
  Logical Operator13/1 -> Logical Operator11/1
  Subsystem3/1(Out1) -> Out4/1
  In2/1 -> Subsystem6/1(In1), Subsystem5/1(In1)
  Logical Operator6/1 -> Logical Operator7/3
  Subsystem6/1(Out1) -> Logical Operator13/4, Logical Operator12/3, Logical Operator9/2, Logical Operator6/2, Logical Operator8/4, Logical Operator5/3
  Logical Operator7/1 -> Subsystem7/3(In3)
  Subsystem1/2(Out2) -> Logical Operator12/1, Logical Operator3/1, Logical Operator1/2, Logical Operator5/1
  In5/1 -> Subsystem2/3(In3), Logical Operator13/1, Logical Operator8/1, Logical Operator2/1, Logical Operator/2
  In4/1 -> Subsystem2/1(In1), Subsystem1/1(In1)
  Subsystem8/1(Out1) -> Logical Operator13/5, Logical Operator12/4, Logical Operator10/2, Logical Operator9/3
  Subsystem7/1(Out1) -> Out2/1
  Subsystem4/2(Out2) -> Logical Operator9/1, Logical Operator6/1, Logical Operator4/3
  Logical Operator4/1 -> Subsystem5/3(In3)
  Logical Operator1/1 -> Subsystem3/3(In3)

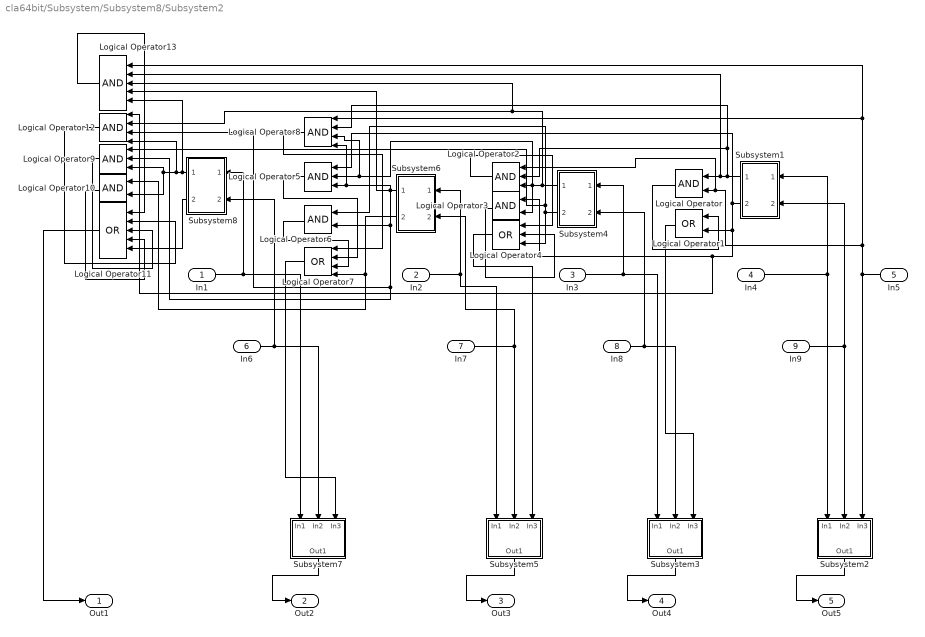
== system cla64bit/Subsystem/Subsystem8/Subsystem2 ==
  In1 : Inport
  In2 : Inport  Port=2
  In3 : Inport  Port=3
  In4 : Inport  Port=4
  In5 : Inport  Port=5
  In6 : Inport  Port=6
  In7 : Inport  Port=7
  In8 : Inport  Port=8
  In9 : Inport  Port=9
  Logical Operator{,3,6,10} (4 alike) : Logic  AllPortsSameDT=off  OutDataTypeStr=boolean
  Logical Operator1 : Logic  Operator=OR  AllPortsSameDT=off  OutDataTypeStr=boolean
  Logical Operator11 : Logic  Operator=OR  Inputs=5  AllPortsSameDT=off  OutDataTypeStr=boolean
  Logical Operator12 : Logic  Inputs=4  AllPortsSameDT=off  OutDataTypeStr=boolean
  Logical Operator13 : Logic  Inputs=5  AllPortsSameDT=off  OutDataTypeStr=boolean
  Logical Operator2 : Logic  Inputs=3  AllPortsSameDT=off  OutDataTypeStr=boolean
  Logical Operator4 : Logic  Operator=OR  Inputs=3  AllPortsSameDT=off  OutDataTypeStr=boolean
  Logical Operator5 : Logic  Inputs=3  AllPortsSameDT=off  OutDataTypeStr=boolean
  Logical Operator7 : Logic  Operator=OR  Inputs=4  AllPortsSameDT=off  OutDataTypeStr=boolean
  Logical Operator8 : Logic  Inputs=4  AllPortsSameDT=off  OutDataTypeStr=boolean
  Logical Operator9 : Logic  Inputs=3  AllPortsSameDT=off  OutDataTypeStr=boolean
  Subsystem1 : Subsystem
  Subsystem2 : Subsystem
  Subsystem3 : Subsystem
  Subsystem4 : Subsystem
  Subsystem5 : Subsystem
  Subsystem6 : Subsystem
  Subsystem7 : Subsystem
  Subsystem8 : Subsystem
  Out1 : Outport
  Out2 : Outport  Port=2
  Out3 : Outport  Port=3
  Out4 : Outport  Port=4
  Out5 : Outport  Port=5
  wires:
  Subsystem8/2(Out2) -> Logical Operator11/5
  Subsystem5/1(Out1) -> Out3/1
  Logical Operator8/1 -> Logical Operator7/1
  Logical Operator9/1 -> Logical Operator11/3
  Logical Operator5/1 -> Logical Operator7/2
  Logical Operator10/1 -> Logical Operator11/4
  Logical Operator3/1 -> Logical Operator4/2
  Logical Operator/1 -> Logical Operator1/1
  In3/1 -> Subsystem3/1(In1), Subsystem4/1(In1)
  Subsystem6/2(Out2) -> Logical Operator10/1, Logical Operator7/4
  Logical Operator12/1 -> Logical Operator11/2
  In7/1 -> Subsystem5/2(In2), Subsystem6/2(In2)
  Subsystem2/1(Out1) -> Out5/1
  In1/1 -> Subsystem8/1(In1), Subsystem7/1(In1)
  In6/1 -> Subsystem7/2(In2), Subsystem8/2(In2)
  Subsystem1/1(Out1) -> Logical Operator8/2, Logical Operator2/2, Logical Operator13/2, Logical Operator/1
  In9/1 -> Subsystem2/2(In2), Subsystem1/2(In2)
  In8/1 -> Subsystem3/2(In2), Subsystem4/2(In2)
  Logical Operator11/1 -> Out1/1
  Logical Operator2/1 -> Logical Operator4/1
  Subsystem4/1(Out1) -> Logical Operator8/3, Logical Operator5/2, Logical Operator3/2, Logical Operator2/3, Logical Operator13/3, Logical Operator12/2
  Logical Operator13/1 -> Logical Operator11/1
  Subsystem3/1(Out1) -> Out4/1
  In2/1 -> Subsystem6/1(In1), Subsystem5/1(In1)
  Logical Operator6/1 -> Logical Operator7/3
  Subsystem6/1(Out1) -> Logical Operator13/4, Logical Operator12/3, Logical Operator9/2, Logical Operator6/2, Logical Operator8/4, Logical Operator5/3
  Logical Operator7/1 -> Subsystem7/3(In3)
  Subsystem1/2(Out2) -> Logical Operator12/1, Logical Operator3/1, Logical Operator1/2, Logical Operator5/1
  In5/1 -> Subsystem2/3(In3), Logical Operator13/1, Logical Operator8/1, Logical Operator2/1, Logical Operator/2
  In4/1 -> Subsystem2/1(In1), Subsystem1/1(In1)
  Subsystem8/1(Out1) -> Logical Operator13/5, Logical Operator12/4, Logical Operator10/2, Logical Operator9/3
  Subsystem7/1(Out1) -> Out2/1
  Subsystem4/2(Out2) -> Logical Operator9/1, Logical Operator6/1, Logical Operator4/3
  Logical Operator4/1 -> Subsystem5/3(In3)
  Logical Operator1/1 -> Subsystem3/3(In3)
